simulink model "PD_Diagonal"  (R2015a)
settings: Solver=ode4  StartTime=0.0  StopTime=15  RelTol=1e-3
model workspace: external: MAT-File co-effs.mat (data not in the file)
undefined symbols (not defined in the file or in its folder): magnitude
libraries: aerolibutil x104, vrlib x5, dspmathops x4, simulink_extras x2, simulink x1, dspinverses x1
(part 2 of 3)

== system PD_Diagonal/M2/M2->B Transformation ==
  note: X->Y->Z Transformation Sequence M2->B
  X : Inport
  Y : Inport  Port=2
  "Z " : Inport  Port=3
  Quaternion Multiplication : aerolibutil/Quaternion Multiplication
  Quaternion Multiplication1 : aerolibutil/Quaternion Multiplication
  X Quaternion : Subsystem
  Y Quaternion : Subsystem
  Z Quaternion : Subsystem
  Q_m2 : Outport
  tag scope: M2x=global, M2y=global, M2z=global
  wires:
  X/1 -> X Quaternion/1(y(X Rad)), [M2x]
  "Z "/1 -> [M2z], Z Quaternion/1(Z Rad)
  Y/1 -> Y Quaternion/1(h(Y Rad)), [M2y]
  Y Quaternion/1(Q_y) -> Quaternion Multiplication/2  "Qy"
  X Quaternion/1(Q_x) -> Quaternion Multiplication/1  "Qx"
  Quaternion Multiplication/1 -> Quaternion Multiplication1/1  "Qx*Qy"
  Z Quaternion/1(Q_z) -> Quaternion Multiplication1/2  "Qz"
  Quaternion Multiplication1/1 -> Q_m2/1  "Qx*Qy*Qz"

== system PD_Diagonal/M3/M3 DC Motor ==
  note: M3 DC Motor response
  Set Speed(rpm) : Inport
  ->ms : Product  Inputs=*/
  10080 Max : Saturate  UpperLimit=10080  LowerLimit=-10080
  Add : Sum
  Dead Time (ms) : Constant
  Dead Time Block : VariableTransportDelay  MaximumDelay=10
  Miliseconds : Constant  Value=1000
  Starting Speed : Constant  Value=10080
  Subtract : Sum  Inputs=+-
  Transfer Fcn : TransferFcn  Numerator=1  Denominator=[0.6 1]
  Speed (rpm) : Outport
  wires:
  Dead Time Block/1 -> Transfer Fcn/1
  Miliseconds/1 -> ->ms/2
  Dead Time (ms)/1 -> ->ms/1
  ->ms/1 -> Dead Time Block/2
  Transfer Fcn/1 -> 10080 Max/1
  Set Speed(rpm)/1 -> Subtract/1
  10080 Max/1 -> Add/1
  Add/1 -> Speed (rpm)/1
  Starting Speed/1 -> Subtract/2, Add/2
  Subtract/1 -> Dead Time Block/1

== system PD_Diagonal/M3/M3 Speed to Thrust ==
  note: RPS to Thrust
  Speed(RPM) : Inport
  ->RPS : Product  Inputs=*/
  Force Coefficient CT : Constant  Value=0.000243
  M1 w^2 : Math  Operator=magnitude^2  SaturateOnIntegerOverflow=on
  Mins : Constant  Value=60
  Product : Product
  Thrust(N) : Outport
  wires:
  M1 w^2/1 -> Product/2
  ->RPS/1 -> M1 w^2/1
  Speed(RPM)/1 -> ->RPS/1
  Force Coefficient CT/1 -> Product/1
  Mins/1 -> ->RPS/2
  Product/1 -> Thrust(N)/1

== system PD_Diagonal/M3/M3 X Servo  ==
  note: 0V Servo = 0 degree / +90 offset
      | 2.5v Servo = 90 degree/ 0 offset
      | 5v Servo = 180 degree / -90 offset
  note: Servo zero position = 2.5v = 90 degree vertical
  note: 2.5v = 90 degree
  note: 2.5v = 0 offset
  note: M3X Servo Response v->rad
  Input(v) : Inport
  ->ms : Product  Inputs=*/
  ->rad : Constant  Value=pi/5
  Add : Sum  Inputs=+-
  Dead Time (ms) : Constant  Value=3
  Dead Time Block : VariableTransportDelay  MaximumDelay=10  MaximumPoints=2048
  Default Zero : Constant  Value=pi/2
  Divide : Product  Inputs=*/
  Miliseconds : Constant  Value=1000
  Multiply : Product  Inputs=**
  Saturation : Subsystem
  Scope : Scope
      settings: SaveName=ScopeData3
  Starting Position(v) : Constant  Value=2.5
  Subtract : Sum  Inputs=|-+
  Subtract1 : Sum  Inputs=+-|
  Supply (V) : Constant  Value=5
  Transfer Fcn : TransferFcn  Numerator=[pi]  Denominator=[0.11 1]
  Position (rad) : Outport
  wires:
  Miliseconds/1 -> ->ms/2
  Dead Time (ms)/1 -> ->ms/1
  Supply (V)/1 -> Divide/2
  Divide/1 -> Dead Time Block/1
  ->ms/1 -> Dead Time Block/2  "Deadtime 3ms (333hz digital)"
  Dead Time Block/1 -> Transfer Fcn/1
  ->rad/1 -> Multiply/2
  Transfer Fcn/1 -> Saturation/1(Rad)
  Saturation/1(Out1) -> Add/1
  [Lim] -> Saturation/2(1/0)
  Starting Position(v)/1 -> Multiply/1, Subtract/2
  Subtract/1 -> Divide/1
  Add/1 -> Scope/1, Position (rad)/1
  Multiply/1 -> Subtract1/2
  Input(v)/1 -> Subtract/1
  Subtract1/1 -> Add/2
  Default Zero/1 -> Subtract1/1

== system PD_Diagonal/M3/M3 Y Servo ==
  note: 0V Servo = 0 degree / +90 offset
      | 2.5v Servo = 90 degree/ 0 offset
      | 5v Servo = 180 degree / -90 offset
  note: Servo zero position = 2.5v = 90 degree vertical
  note: 2.5v = 90 degree
  note: 2.5v = 0 offset
  note: M3Y Servo Response v->rad
  Input(v) : Inport
  ->ms : Product  Inputs=*/
  ->rad : Constant  Value=pi/5
  Add : Sum  Inputs=+-
  Dead Time (ms) : Constant  Value=3
  Dead Time Block : VariableTransportDelay  MaximumDelay=10  MaximumPoints=2048
  Default Zero : Constant  Value=pi/2
  Divide : Product  Inputs=*/
  Miliseconds : Constant  Value=1000
  Multiply : Product  Inputs=**
  Saturation : Subsystem
  Scope : Scope
      settings: SaveName=ScopeData4
  Starting Position(v) : Constant  Value=2.5
  Subtract : Sum  Inputs=|-+
  Subtract1 : Sum  Inputs=+-|
  Supply (V) : Constant  Value=5
  Transfer Fcn : TransferFcn  Numerator=[pi]  Denominator=[0.11 1]
  Position (rad) : Outport
  wires:
  Miliseconds/1 -> ->ms/2
  Dead Time (ms)/1 -> ->ms/1
  Supply (V)/1 -> Divide/2
  Divide/1 -> Dead Time Block/1
  ->ms/1 -> Dead Time Block/2  "Deadtime 3ms (333hz digital)"
  Dead Time Block/1 -> Transfer Fcn/1
  ->rad/1 -> Multiply/2
  Transfer Fcn/1 -> Saturation/1(Rad)
  Saturation/1(Out1) -> Add/1
  [Lim] -> Saturation/2(1/0)
  Starting Position(v)/1 -> Multiply/1, Subtract/2
  Subtract/1 -> Divide/1
  Add/1 -> Scope/1, Position (rad)/1
  Multiply/1 -> Subtract1/2
  Input(v)/1 -> Subtract/1
  Subtract1/1 -> Add/2
  Default Zero/1 -> Subtract1/1

== system PD_Diagonal/M3/M3->B Transformation ==
  note: X->Y->Z Transformation Sequence M3->B
  X : Inport
  Y : Inport  Port=2
  "Z " : Inport  Port=3
  Quaternion Multiplication : aerolibutil/Quaternion Multiplication
  Quaternion Multiplication1 : aerolibutil/Quaternion Multiplication
  X Quaternion : Subsystem
  Y Quaternion : Subsystem
  Z Quaternion : Subsystem
  Q_m3 : Outport
  tag scope: M3x=global, M3y=global, M3z=global
  wires:
  X/1 -> X Quaternion/1(y(X Rad)), [M3x]
  "Z "/1 -> [M3z], Z Quaternion/1(Z Rad)
  Y/1 -> Y Quaternion/1(h(Y Rad)), [M3y]
  Y Quaternion/1(Q_y) -> Quaternion Multiplication/2  "Qy"
  X Quaternion/1(Q_x) -> Quaternion Multiplication/1  "Qx"
  Quaternion Multiplication/1 -> Quaternion Multiplication1/1  "Qx*Qy"
  Z Quaternion/1(Q_z) -> Quaternion Multiplication1/2  "Qz"
  Quaternion Multiplication1/1 -> Q_m3/1  "Qx*Qy*Qz"

== system PD_Diagonal/M4/M4 DC Motor ==
  note: M4 DC Motor response
  Set Speed(rpm) : Inport
  ->ms : Product  Inputs=*/
  10080 Max : Saturate  UpperLimit=10080  LowerLimit=-10080
  Add : Sum
  Dead Time (ms) : Constant
  Dead Time Block : VariableTransportDelay  MaximumDelay=10
  Miliseconds : Constant  Value=1000
  Starting Speed : Constant  Value=-10080
  Subtract : Sum  Inputs=+-
  Transfer Fcn : TransferFcn  Numerator=1  Denominator=[0.6 1]
  Speed (rpm) : Outport
  wires:
  Dead Time Block/1 -> Transfer Fcn/1
  Miliseconds/1 -> ->ms/2
  Dead Time (ms)/1 -> ->ms/1
  ->ms/1 -> Dead Time Block/2
  Transfer Fcn/1 -> 10080 Max/1
  Set Speed(rpm)/1 -> Subtract/1
  10080 Max/1 -> Add/1
  Add/1 -> Speed (rpm)/1
  Starting Speed/1 -> Subtract/2, Add/2
  Subtract/1 -> Dead Time Block/1

== system PD_Diagonal/M4/M4 Speed to Thrust ==
  note: RPS to Thrust
  Speed(RPM) : Inport
  ->RPS : Product  Inputs=*/
  Force Coefficient CT : Constant  Value=0.000243
  M1 w^2 : Math  Operator=magnitude^2  SaturateOnIntegerOverflow=on
  Mins : Constant  Value=60
  Product : Product
  Thrust(N) : Outport
  wires:
  M1 w^2/1 -> Product/2
  ->RPS/1 -> M1 w^2/1
  Speed(RPM)/1 -> ->RPS/1
  Force Coefficient CT/1 -> Product/1
  Mins/1 -> ->RPS/2
  Product/1 -> Thrust(N)/1

== system PD_Diagonal/M4/M4 X Servo  ==
  note: 0V Servo = 0 degree / +90 offset
      | 2.5v Servo = 90 degree/ 0 offset
      | 5v Servo = 180 degree / -90 offset
  note: Servo zero position = 2.5v = 90 degree vertical
  note: 2.5v = 90 degree
  note: 2.5v = 0 offset
  note: M4X Servo Response v->rad
  Input(v) : Inport
  ->ms : Product  Inputs=*/
  ->rad : Constant  Value=pi/5
  Add : Sum  Inputs=+-
  Dead Time (ms) : Constant  Value=3
  Dead Time Block : VariableTransportDelay  MaximumDelay=10  MaximumPoints=2048
  Default Zero : Constant  Value=pi/2
  Divide : Product  Inputs=*/
  Miliseconds : Constant  Value=1000
  Multiply : Product  Inputs=**
  Saturation : Subsystem
  Scope : Scope
      settings: SaveName=ScopeData3
  Starting Position(v) : Constant  Value=2.5
  Subtract : Sum  Inputs=|-+
  Subtract1 : Sum  Inputs=+-|
  Supply (V) : Constant  Value=5
  Transfer Fcn : TransferFcn  Numerator=[pi]  Denominator=[0.11 1]
  Position (rad) : Outport
  wires:
  Miliseconds/1 -> ->ms/2
  Dead Time (ms)/1 -> ->ms/1
  Supply (V)/1 -> Divide/2
  Divide/1 -> Dead Time Block/1
  ->ms/1 -> Dead Time Block/2  "Deadtime 3ms (333hz digital)"
  Dead Time Block/1 -> Transfer Fcn/1
  ->rad/1 -> Multiply/2
  Transfer Fcn/1 -> Saturation/1(Rad)
  Saturation/1(Out1) -> Add/1
  [Lim] -> Saturation/2(1/0)
  Starting Position(v)/1 -> Multiply/1, Subtract/2
  Subtract/1 -> Divide/1
  Add/1 -> Scope/1, Position (rad)/1
  Multiply/1 -> Subtract1/2
  Input(v)/1 -> Subtract/1
  Subtract1/1 -> Add/2
  Default Zero/1 -> Subtract1/1

== system PD_Diagonal/M4/M4 Y Servo ==
  note: 0V Servo = 0 degree / +90 offset
      | 2.5v Servo = 90 degree/ 0 offset
      | 5v Servo = 180 degree / -90 offset
  note: Servo zero position = 2.5v = 90 degree vertical
  note: 2.5v = 90 degree
  note: 2.5v = 0 offset
  note: M4Y Servo Response v->rad
  Input(v) : Inport
  ->ms : Product  Inputs=*/
  ->rad : Constant  Value=pi/5
  Add : Sum  Inputs=+-
  Dead Time (ms) : Constant  Value=3
  Dead Time Block : VariableTransportDelay  MaximumDelay=10  MaximumPoints=2048
  Default Zero : Constant  Value=pi/2
  Divide : Product  Inputs=*/
  Miliseconds : Constant  Value=1000
  Multiply : Product  Inputs=**
  Saturation : Subsystem
  Scope : Scope
      settings: SaveName=ScopeData4
  Starting Position(v) : Constant  Value=2.5
  Subtract : Sum  Inputs=|-+
  Subtract1 : Sum  Inputs=+-|
  Supply (V) : Constant  Value=5
  Transfer Fcn : TransferFcn  Numerator=[pi]  Denominator=[0.11 1]
  Position (rad) : Outport
  wires:
  Miliseconds/1 -> ->ms/2
  Dead Time (ms)/1 -> ->ms/1
  Supply (V)/1 -> Divide/2
  Divide/1 -> Dead Time Block/1
  ->ms/1 -> Dead Time Block/2  "Deadtime 3ms (333hz digital)"
  Dead Time Block/1 -> Transfer Fcn/1
  ->rad/1 -> Multiply/2
  Transfer Fcn/1 -> Saturation/1(Rad)
  Saturation/1(Out1) -> Add/1
  [Lim] -> Saturation/2(1/0)
  Starting Position(v)/1 -> Multiply/1, Subtract/2
  Subtract/1 -> Divide/1
  Add/1 -> Scope/1, Position (rad)/1
  Multiply/1 -> Subtract1/2
  Input(v)/1 -> Subtract/1
  Subtract1/1 -> Add/2
  Default Zero/1 -> Subtract1/1

== system PD_Diagonal/M4/M4->B Transformation ==
  note: X->Y->Z Transformation Sequence M4->B
  X : Inport
  Y : Inport  Port=2
  "Z " : Inport  Port=3
  Quaternion Multiplication : aerolibutil/Quaternion Multiplication
  Quaternion Multiplication1 : aerolibutil/Quaternion Multiplication
  X Quaternion : Subsystem
  Y Quaternion : Subsystem
  Z Quaternion : Subsystem
  Q_m4 : Outport
  tag scope: M4x=global, M4y=global, M4z=global
  wires:
  X/1 -> X Quaternion/1(y(X Rad)), [M4x]
  Y/1 -> Y Quaternion/1(h(Y Rad)), [M4y]
  Y Quaternion/1(Q_y) -> Quaternion Multiplication/2  "Qy"
  X Quaternion/1(Q_x) -> Quaternion Multiplication/1  "Qx"
  Quaternion Multiplication/1 -> Quaternion Multiplication1/1  "Qx*Qy"
  Z Quaternion/1(Q_z) -> Quaternion Multiplication1/2  "Qz"
  Quaternion Multiplication1/1 -> Q_m4/1  "Qx*Qy*Qz"
  "Z "/1 -> [M4z], Z Quaternion/1(Z Rad)

== system PD_Diagonal/Quat Error/QuatMultiply1 ==
  Q1 in : Inport  PortDimensions=[4]
  Q2 in : Inport  Port=2  PortDimensions=[4]
  Q1 scalar : Selector  InputPortWidth=4  Indices=[1]
  Q1 vector : Selector  InputPortWidth=4  Indices=[2 3 4]
  Q1.Q2 : DotProduct  InputSameDT=on  OutDataTypeStr=Inherit: Inherit via internal rule
  Q1XQ2 : vrlib/Utilities/Cross Product
  Q2 scalar : Selector  InputPortWidth=4  Indices=[1]
  Q2 vector : Selector  InputPortWidth=4  Indices=[2 3 4]
  Qout scalar : Sum  Inputs=+-
  Qout vector : Sum  Inputs=+++
  Vector Concatenate : Concatenate
  q1.Q2 : Product
  q1.q2 : Product
  q2.Q1 : Product
  Qout : Outport  PortDimensions=[4]
  wires:
  Q1 in/1 -> Q1 vector/1, Q1 scalar/1
  Q2 in/1 -> Q2 vector/1, Q2 scalar/1
  Q1 scalar/1 -> q1.q2/1, q1.Q2/1
  Q2 scalar/1 -> q1.q2/2, q2.Q1/2
  Q1 vector/1 -> Q1.Q2/1, Q1XQ2/1, q2.Q1/1
  Q2 vector/1 -> Q1.Q2/2, Q1XQ2/2, q1.Q2/2
  q1.q2/1 -> Qout scalar/1
  Q1.Q2/1 -> Qout scalar/2
  q2.Q1/1 -> Qout vector/1
  q1.Q2/1 -> Qout vector/2
  Qout scalar/1 -> Vector Concatenate/1
  Qout vector/1 -> Vector Concatenate/2
  Vector Concatenate/1 -> Qout/1
  Q1XQ2/1 -> Qout vector/3  "Q1XQ2"

== system PD_Diagonal/R->Q/QuatMultiply ==
  Q1 in : Inport  PortDimensions=[4]
  Q2 in : Inport  Port=2  PortDimensions=[4]
  Q1 scalar : Selector  InputPortWidth=4  Indices=[1]
  Q1 vector : Selector  InputPortWidth=4  Indices=[2 3 4]
  Q1.Q2 : DotProduct  InputSameDT=on  OutDataTypeStr=Inherit: Inherit via internal rule
  Q1XQ2 : vrlib/Utilities/Cross Product
  Q2 scalar : Selector  InputPortWidth=4  Indices=[1]
  Q2 vector : Selector  InputPortWidth=4  Indices=[2 3 4]
  Qout scalar : Sum  Inputs=+-
  Qout vector : Sum  Inputs=+++
  Vector Concatenate : Concatenate
  q1.Q2 : Product
  q1.q2 : Product
  q2.Q1 : Product
  Qout : Outport  PortDimensions=[4]
  wires:
  Q1 in/1 -> Q1 vector/1, Q1 scalar/1
  Q2 in/1 -> Q2 vector/1, Q2 scalar/1
  Q1 scalar/1 -> q1.q2/1, q1.Q2/1
  Q2 scalar/1 -> q1.q2/2, q2.Q1/2
  Q1 vector/1 -> Q1.Q2/1, q2.Q1/1, Q1XQ2/1
  Q2 vector/1 -> Q1.Q2/2, q1.Q2/2, Q1XQ2/2
  q1.q2/1 -> Qout scalar/1
  Q1.Q2/1 -> Qout scalar/2
  q2.Q1/1 -> Qout vector/1
  q1.Q2/1 -> Qout vector/2
  Q1XQ2/1 -> Qout vector/3
  Qout scalar/1 -> Vector Concatenate/1
  Qout vector/1 -> Vector Concatenate/2
  Vector Concatenate/1 -> Qout/1

== system PD_Diagonal/R->Q/QuatMultiply1 ==
  Q1 in : Inport  PortDimensions=[4]
  Q2 in : Inport  Port=2  PortDimensions=[4]
  Q1 scalar : Selector  InputPortWidth=4  Indices=[1]
  Q1 vector : Selector  InputPortWidth=4  Indices=[2 3 4]
  Q1.Q2 : DotProduct  InputSameDT=on  OutDataTypeStr=Inherit: Inherit via internal rule
  Q1XQ2 : vrlib/Utilities/Cross Product
  Q2 scalar : Selector  InputPortWidth=4  Indices=[1]
  Q2 vector : Selector  InputPortWidth=4  Indices=[2 3 4]
  Qout scalar : Sum  Inputs=+-
  Qout vector : Sum  Inputs=+++
  Vector Concatenate : Concatenate
  q1.Q2 : Product
  q1.q2 : Product
  q2.Q1 : Product
  Qout : Outport  PortDimensions=[4]
  wires:
  Q1 in/1 -> Q1 vector/1, Q1 scalar/1
  Q2 in/1 -> Q2 vector/1, Q2 scalar/1
  Q1 scalar/1 -> q1.q2/1, q1.Q2/1
  Q2 scalar/1 -> q1.q2/2, q2.Q1/2
  Q1 vector/1 -> Q1.Q2/1, Q1XQ2/1, q2.Q1/1
  Q2 vector/1 -> Q1.Q2/2, Q1XQ2/2, q1.Q2/2
  q1.q2/1 -> Qout scalar/1
  Q1.Q2/1 -> Qout scalar/2
  q2.Q1/1 -> Qout vector/1
  q1.Q2/1 -> Qout vector/2
  Qout scalar/1 -> Vector Concatenate/1
  Qout vector/1 -> Vector Concatenate/2
  Vector Concatenate/1 -> Qout/1
  Q1XQ2/1 -> Qout vector/3  "Q1XQ2"

== system PD_Diagonal/Rb0->Q0/QuatMultiply ==
  Q1 in : Inport  PortDimensions=[4]
  Q2 in : Inport  Port=2  PortDimensions=[4]
  Q1 scalar : Selector  InputPortWidth=4  Indices=[1]
  Q1 vector : Selector  InputPortWidth=4  Indices=[2 3 4]
  Q1.Q2 : DotProduct  InputSameDT=on  OutDataTypeStr=Inherit: Inherit via internal rule
  Q1XQ2 : vrlib/Utilities/Cross Product
  Q2 scalar : Selector  InputPortWidth=4  Indices=[1]
  Q2 vector : Selector  InputPortWidth=4  Indices=[2 3 4]
  Qout scalar : Sum  Inputs=+-
  Qout vector : Sum  Inputs=+++
  Vector Concatenate : Concatenate
  q1.Q2 : Product
  q1.q2 : Product
  q2.Q1 : Product
  Qout : Outport  PortDimensions=[4]
  wires:
  Q1 in/1 -> Q1 vector/1, Q1 scalar/1
  Q2 in/1 -> Q2 vector/1, Q2 scalar/1
  Q1 scalar/1 -> q1.q2/1, q1.Q2/1
  Q2 scalar/1 -> q1.q2/2, q2.Q1/2
  Q1 vector/1 -> Q1.Q2/1, q2.Q1/1, Q1XQ2/1
  Q2 vector/1 -> Q1.Q2/2, q1.Q2/2, Q1XQ2/2
  q1.q2/1 -> Qout scalar/1
  Q1.Q2/1 -> Qout scalar/2
  q2.Q1/1 -> Qout vector/1
  q1.Q2/1 -> Qout vector/2
  Q1XQ2/1 -> Qout vector/3
  Qout scalar/1 -> Vector Concatenate/1
  Qout vector/1 -> Vector Concatenate/2
  Vector Concatenate/1 -> Qout/1

== system PD_Diagonal/Rb0->Q0/QuatMultiply1 ==
  Q1 in : Inport  PortDimensions=[4]
  Q2 in : Inport  Port=2  PortDimensions=[4]
  Q1 scalar : Selector  InputPortWidth=4  Indices=[1]
  Q1 vector : Selector  InputPortWidth=4  Indices=[2 3 4]
  Q1.Q2 : DotProduct  InputSameDT=on  OutDataTypeStr=Inherit: Inherit via internal rule
  Q1XQ2 : vrlib/Utilities/Cross Product
  Q2 scalar : Selector  InputPortWidth=4  Indices=[1]
  Q2 vector : Selector  InputPortWidth=4  Indices=[2 3 4]
  Qout scalar : Sum  Inputs=+-
  Qout vector : Sum  Inputs=+++
  Vector Concatenate : Concatenate
  q1.Q2 : Product
  q1.q2 : Product
  q2.Q1 : Product
  Qout : Outport  PortDimensions=[4]
  wires:
  Q1 in/1 -> Q1 vector/1, Q1 scalar/1
  Q2 in/1 -> Q2 vector/1, Q2 scalar/1
  Q1 scalar/1 -> q1.q2/1, q1.Q2/1
  Q2 scalar/1 -> q1.q2/2, q2.Q1/2
  Q1 vector/1 -> Q1.Q2/1, Q1XQ2/1, q2.Q1/1
  Q2 vector/1 -> Q1.Q2/2, Q1XQ2/2, q1.Q2/2
  q1.q2/1 -> Qout scalar/1
  Q1.Q2/1 -> Qout scalar/2
  q2.Q1/1 -> Qout vector/1
  q1.Q2/1 -> Qout vector/2
  Qout scalar/1 -> Vector Concatenate/1
  Qout vector/1 -> Vector Concatenate/2
  Vector Concatenate/1 -> Qout/1
  Q1XQ2/1 -> Qout vector/3  "Q1XQ2"

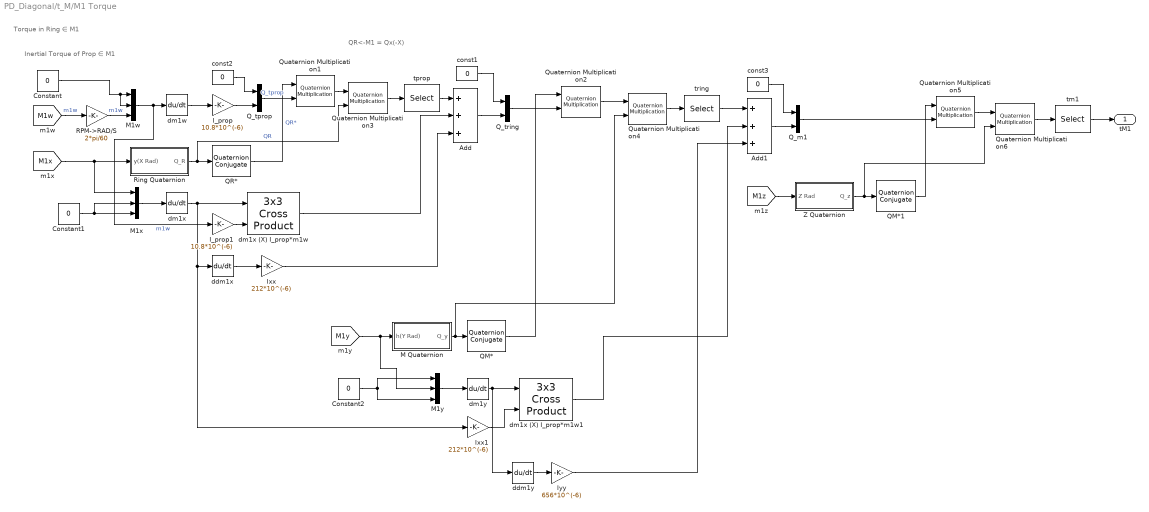
== system PD_Diagonal/t_M/M1 Torque ==
  note: QR<-M1 = Qx(-X)
  note: Torque in Ring ∈ M1
  note: Inertial Torque of Prop ∈ M1
  Add : Sum  Inputs=+++
  Add1 : Sum  Inputs=+++
  Constant : Constant  Value=0
  Constant1 : Constant  Value=0
  Constant2 : Constant  Value=0
  I_prop : Gain  Gain=10.8*10^(-6)
  I_prop1 : Gain  Gain=10.8*10^(-6)
  Ixx : Gain  Gain=212*10^(-6)
  Ixx1 : Gain  Gain=212*10^(-6)
  Iyy : Gain  Gain=656*10^(-6)
  M Quaternion : Subsystem
  M1w : Concatenate  NumInputs=3
  M1x : Concatenate  NumInputs=3
  M1y : Concatenate  NumInputs=3
  QM* : aerolibutil/Quaternion Conjugate
  QM*1 : aerolibutil/Quaternion Conjugate
  QR* : aerolibutil/Quaternion Conjugate
  Q_m1 : Concatenate
  Q_tprop : Concatenate
  Q_tring : Concatenate
  Quaternion Multiplication{1..6} (6 alike) : aerolibutil/Quaternion Multiplication
  RPM->RAD/S : Gain  Gain=2*pi/60
  Ring Quaternion : Subsystem
  Z Quaternion : Subsystem
  const1 : Constant  Value=0
  const2 : Constant  Value=0
  const3 : Constant  Value=0
  ddm1x : Derivative
  ddm1y : Derivative
  dm1w : Derivative
  dm1x : Derivative
  dm1x (X) I_prop*m1w : aerolibutil/3x3 Cross Product
  dm1x (X) I_prop*m1w1 : aerolibutil/3x3 Cross Product
  dm1y : Derivative
  tm1 : Selector  InputPortWidth=4  Indices=[2 3 4]
  tprop : Selector  InputPortWidth=4  Indices=[2 3 4]
  tring : Selector  InputPortWidth=4  Indices=[2 3 4]
  tM1 : Outport
  wires:
  [M1w] -> RPM->RAD/S/1  "m1w"
  RPM->RAD/S/1 -> M1w/3  "m1w"
  Constant/1 -> M1w/2, M1w/1
  dm1w/1 -> I_prop/1
  [M1x] -> M1x/1, Ring Quaternion/1(y(X Rad))
  Ring Quaternion/1(Q_R) -> Quaternion Multiplication3/2, QR*/1  "QR"
  const2/1 -> Q_tprop/1
  Quaternion Multiplication1/1 -> Quaternion Multiplication3/1
  Q_tprop/1 -> Quaternion Multiplication1/2  "Q_tprop"
  QR*/1 -> Quaternion Multiplication1/1  "QR*"
  I_prop/1 -> Q_tprop/2
  dm1x/1 -> Ixx1/1, ddm1x/1, dm1x (X) I_prop*m1w/1
  I_prop1/1 -> dm1x (X) I_prop*m1w/2
  dm1x (X) I_prop*m1w/1 -> Add/2
  M1w/1 -> I_prop1/1, dm1w/1  "m1w"
  M1x/1 -> dm1x/1
  ddm1x/1 -> Ixx/1
  Ixx/1 -> Add/3
  Quaternion Multiplication3/1 -> tprop/1
  tprop/1 -> Add/1
  [M1y] -> M1y/2, M Quaternion/1(h(Y Rad))
  const1/1 -> Q_tring/1
  Add/1 -> Q_tring/2
  Q_tring/1 -> Quaternion Multiplication2/2
  M Quaternion/1(Q_y) -> Quaternion Multiplication4/2, QM*/1
  QM*/1 -> Quaternion Multiplication2/1
  Quaternion Multiplication2/1 -> Quaternion Multiplication4/1
  Quaternion Multiplication4/1 -> tring/1
  tring/1 -> Add1/1
  Constant1/1 -> M1x/2, M1x/3
  Constant2/1 -> M1y/1, M1y/3
  M1y/1 -> dm1y/1
  Ixx1/1 -> dm1x (X) I_prop*m1w1/2
  dm1x (X) I_prop*m1w1/1 -> Add1/2
  dm1y/1 -> ddm1y/1, dm1x (X) I_prop*m1w1/1
  ddm1y/1 -> Iyy/1
  Iyy/1 -> Add1/3
  [M1z] -> Z Quaternion/1(Z Rad)
  const3/1 -> Q_m1/1
  Add1/1 -> Q_m1/2
  Q_m1/1 -> Quaternion Multiplication5/2
  Z Quaternion/1(Q_z) -> Quaternion Multiplication6/2, QM*1/1
  QM*1/1 -> Quaternion Multiplication5/1
  Quaternion Multiplication5/1 -> Quaternion Multiplication6/1
  Quaternion Multiplication6/1 -> tm1/1
  tm1/1 -> tM1/1

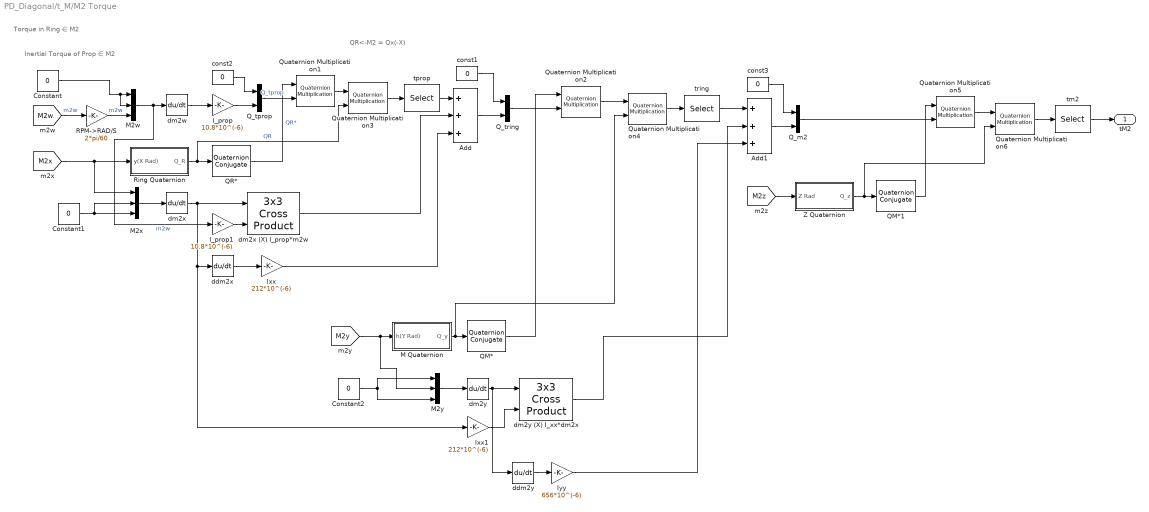
== system PD_Diagonal/t_M/M2 Torque ==
  note: QR<-M2 = Qx(-X)
  note: Torque in Ring ∈ M2
  note: Inertial Torque of Prop ∈ M2
  Add : Sum  Inputs=+++
  Add1 : Sum  Inputs=+++
  Constant : Constant  Value=0
  Constant1 : Constant  Value=0
  Constant2 : Constant  Value=0
  I_prop : Gain  Gain=10.8*10^(-6)
  I_prop1 : Gain  Gain=10.8*10^(-6)
  Ixx : Gain  Gain=212*10^(-6)
  Ixx1 : Gain  Gain=212*10^(-6)
  Iyy : Gain  Gain=656*10^(-6)
  M Quaternion : Subsystem
  M2w : Concatenate  NumInputs=3
  M2x : Concatenate  NumInputs=3
  M2y : Concatenate  NumInputs=3
  QM* : aerolibutil/Quaternion Conjugate
  QM*1 : aerolibutil/Quaternion Conjugate
  QR* : aerolibutil/Quaternion Conjugate
  Q_m2 : Concatenate
  Q_tprop : Concatenate
  Q_tring : Concatenate
  Quaternion Multiplication{1..6} (6 alike) : aerolibutil/Quaternion Multiplication
  RPM->RAD/S : Gain  Gain=2*pi/60
  Ring Quaternion : Subsystem
  Z Quaternion : Subsystem
  const1 : Constant  Value=0
  const2 : Constant  Value=0
  const3 : Constant  Value=0
  ddm2x : Derivative
  ddm2y : Derivative
  dm2w : Derivative
  dm2x : Derivative
  dm2x (X) I_prop*m2w : aerolibutil/3x3 Cross Product
  dm2y : Derivative
  dm2y (X) I_xx*dm2x : aerolibutil/3x3 Cross Product
  tm2 : Selector  InputPortWidth=4  Indices=[2 3 4]
  tprop : Selector  InputPortWidth=4  Indices=[2 3 4]
  tring : Selector  InputPortWidth=4  Indices=[2 3 4]
  tM2 : Outport
  wires:
  [M2w] -> RPM->RAD/S/1  "m2w"
  RPM->RAD/S/1 -> M2w/3  "m2w"
  Constant/1 -> M2w/2, M2w/1
  dm2w/1 -> I_prop/1
  [M2x] -> M2x/1, Ring Quaternion/1(y(X Rad))
  Ring Quaternion/1(Q_R) -> Quaternion Multiplication3/2, QR*/1  "QR"
  const2/1 -> Q_tprop/1
  Quaternion Multiplication1/1 -> Quaternion Multiplication3/1
  Q_tprop/1 -> Quaternion Multiplication1/2  "Q_tprop"
  QR*/1 -> Quaternion Multiplication1/1  "QR*"
  I_prop/1 -> Q_tprop/2
  dm2x/1 -> Ixx1/1, ddm2x/1, dm2x (X) I_prop*m2w/1
  I_prop1/1 -> dm2x (X) I_prop*m2w/2
  dm2x (X) I_prop*m2w/1 -> Add/2
  M2w/1 -> I_prop1/1, dm2w/1  "m2w"
  M2x/1 -> dm2x/1
  ddm2x/1 -> Ixx/1
  Ixx/1 -> Add/3
  Quaternion Multiplication3/1 -> tprop/1
  tprop/1 -> Add/1
  [M2y] -> M2y/2, M Quaternion/1(h(Y Rad))
  const1/1 -> Q_tring/1
  Add/1 -> Q_tring/2
  Q_tring/1 -> Quaternion Multiplication2/2
  M Quaternion/1(Q_y) -> Quaternion Multiplication4/2, QM*/1
  QM*/1 -> Quaternion Multiplication2/1
  Quaternion Multiplication2/1 -> Quaternion Multiplication4/1
  Quaternion Multiplication4/1 -> tring/1
  tring/1 -> Add1/1
  Constant1/1 -> M2x/2, M2x/3
  Constant2/1 -> M2y/1, M2y/3
  M2y/1 -> dm2y/1
  Ixx1/1 -> dm2y (X) I_xx*dm2x/2
  dm2y (X) I_xx*dm2x/1 -> Add1/2
  dm2y/1 -> ddm2y/1, dm2y (X) I_xx*dm2x/1
  ddm2y/1 -> Iyy/1
  Iyy/1 -> Add1/3
  [M2z] -> Z Quaternion/1(Z Rad)
  const3/1 -> Q_m2/1
  Add1/1 -> Q_m2/2
  Q_m2/1 -> Quaternion Multiplication5/2
  Z Quaternion/1(Q_z) -> Quaternion Multiplication6/2, QM*1/1
  QM*1/1 -> Quaternion Multiplication5/1
  Quaternion Multiplication5/1 -> Quaternion Multiplication6/1
  Quaternion Multiplication6/1 -> tm2/1
  tm2/1 -> tM2/1

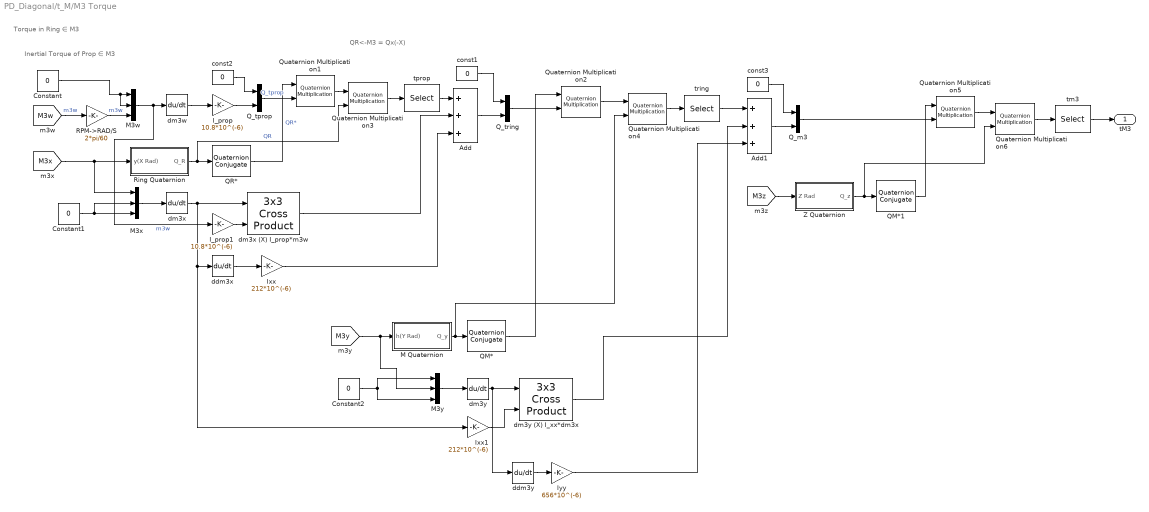
== system PD_Diagonal/t_M/M3 Torque ==
  note: QR<-M3 = Qx(-X)
  note: Torque in Ring ∈ M3
  note: Inertial Torque of Prop ∈ M3
  Add : Sum  Inputs=+++
  Add1 : Sum  Inputs=+++
  Constant : Constant  Value=0
  Constant1 : Constant  Value=0
  Constant2 : Constant  Value=0
  I_prop : Gain  Gain=10.8*10^(-6)
  I_prop1 : Gain  Gain=10.8*10^(-6)
  Ixx : Gain  Gain=212*10^(-6)
  Ixx1 : Gain  Gain=212*10^(-6)
  Iyy : Gain  Gain=656*10^(-6)
  M Quaternion : Subsystem
  M3w : Concatenate  NumInputs=3
  M3x : Concatenate  NumInputs=3
  M3y : Concatenate  NumInputs=3
  QM* : aerolibutil/Quaternion Conjugate
  QM*1 : aerolibutil/Quaternion Conjugate
  QR* : aerolibutil/Quaternion Conjugate
  Q_m3 : Concatenate
  Q_tprop : Concatenate
  Q_tring : Concatenate
  Quaternion Multiplication{1..6} (6 alike) : aerolibutil/Quaternion Multiplication
  RPM->RAD/S : Gain  Gain=2*pi/60
  Ring Quaternion : Subsystem
  Z Quaternion : Subsystem
  const1 : Constant  Value=0
  const2 : Constant  Value=0
  const3 : Constant  Value=0
  ddm3x : Derivative
  ddm3y : Derivative
  dm3w : Derivative
  dm3x : Derivative
  dm3x (X) I_prop*m3w : aerolibutil/3x3 Cross Product
  dm3y : Derivative
  dm3y (X) I_xx*dm3x : aerolibutil/3x3 Cross Product
  tm3 : Selector  InputPortWidth=4  Indices=[2 3 4]
  tprop : Selector  InputPortWidth=4  Indices=[2 3 4]
  tring : Selector  InputPortWidth=4  Indices=[2 3 4]
  tM3 : Outport
  wires:
  [M3w] -> RPM->RAD/S/1  "m3w"
  RPM->RAD/S/1 -> M3w/3  "m3w"
  Constant/1 -> M3w/2, M3w/1
  dm3w/1 -> I_prop/1
  [M3x] -> M3x/1, Ring Quaternion/1(y(X Rad))
  Ring Quaternion/1(Q_R) -> Quaternion Multiplication3/2, QR*/1  "QR"
  const2/1 -> Q_tprop/1
  Quaternion Multiplication1/1 -> Quaternion Multiplication3/1
  Q_tprop/1 -> Quaternion Multiplication1/2  "Q_tprop"
  QR*/1 -> Quaternion Multiplication1/1  "QR*"
  I_prop/1 -> Q_tprop/2
  dm3x/1 -> Ixx1/1, ddm3x/1, dm3x (X) I_prop*m3w/1
  I_prop1/1 -> dm3x (X) I_prop*m3w/2
  dm3x (X) I_prop*m3w/1 -> Add/2
  M3w/1 -> I_prop1/1, dm3w/1  "m3w"
  M3x/1 -> dm3x/1
  ddm3x/1 -> Ixx/1
  Ixx/1 -> Add/3
  Quaternion Multiplication3/1 -> tprop/1
  tprop/1 -> Add/1
  [M3y] -> M3y/2, M Quaternion/1(h(Y Rad))
  const1/1 -> Q_tring/1
  Add/1 -> Q_tring/2
  Q_tring/1 -> Quaternion Multiplication2/2
  M Quaternion/1(Q_y) -> Quaternion Multiplication4/2, QM*/1
  QM*/1 -> Quaternion Multiplication2/1
  Quaternion Multiplication2/1 -> Quaternion Multiplication4/1
  Quaternion Multiplication4/1 -> tring/1
  tring/1 -> Add1/1
  Constant1/1 -> M3x/2, M3x/3
  Constant2/1 -> M3y/1, M3y/3
  M3y/1 -> dm3y/1
  Ixx1/1 -> dm3y (X) I_xx*dm3x/2
  dm3y (X) I_xx*dm3x/1 -> Add1/2
  dm3y/1 -> ddm3y/1, dm3y (X) I_xx*dm3x/1
  ddm3y/1 -> Iyy/1
  Iyy/1 -> Add1/3
  [M3z] -> Z Quaternion/1(Z Rad)
  const3/1 -> Q_m3/1
  Add1/1 -> Q_m3/2
  Q_m3/1 -> Quaternion Multiplication5/2
  Z Quaternion/1(Q_z) -> Quaternion Multiplication6/2, QM*1/1
  QM*1/1 -> Quaternion Multiplication5/1
  Quaternion Multiplication5/1 -> Quaternion Multiplication6/1
  Quaternion Multiplication6/1 -> tm3/1
  tm3/1 -> tM3/1

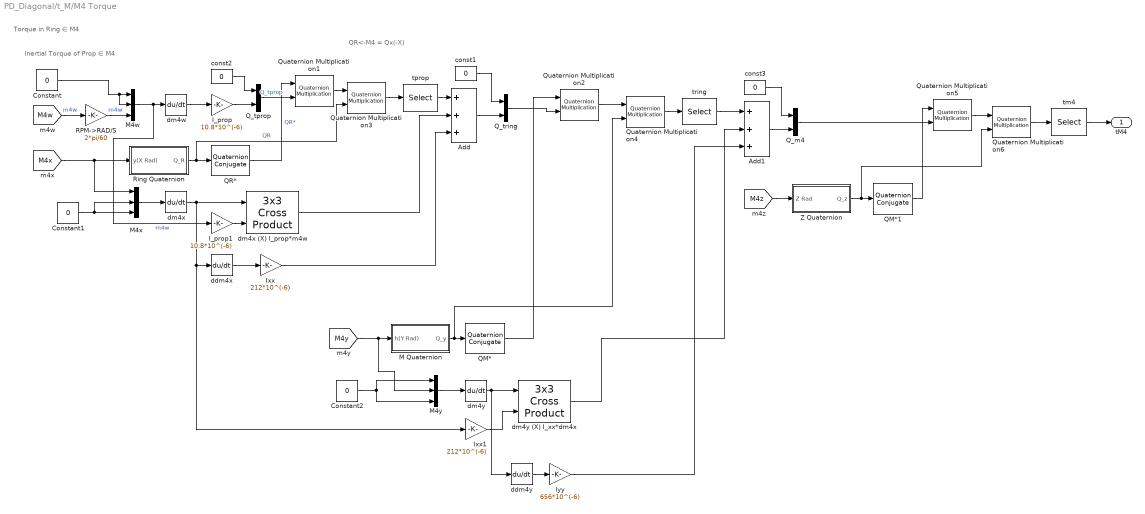
== system PD_Diagonal/t_M/M4 Torque ==
  note: QR<-M4 = Qx(-X)
  note: Torque in Ring ∈ M4
  note: Inertial Torque of Prop ∈ M4
  Add : Sum  Inputs=+++
  Add1 : Sum  Inputs=+++
  Constant : Constant  Value=0
  Constant1 : Constant  Value=0
  Constant2 : Constant  Value=0
  I_prop : Gain  Gain=10.8*10^(-6)
  I_prop1 : Gain  Gain=10.8*10^(-6)
  Ixx : Gain  Gain=212*10^(-6)
  Ixx1 : Gain  Gain=212*10^(-6)
  Iyy : Gain  Gain=656*10^(-6)
  M Quaternion : Subsystem
  M4w : Concatenate  NumInputs=3
  M4x : Concatenate  NumInputs=3
  M4y : Concatenate  NumInputs=3
  QM* : aerolibutil/Quaternion Conjugate
  QM*1 : aerolibutil/Quaternion Conjugate
  QR* : aerolibutil/Quaternion Conjugate
  Q_m4 : Concatenate
  Q_tprop : Concatenate
  Q_tring : Concatenate
  Quaternion Multiplication{1..6} (6 alike) : aerolibutil/Quaternion Multiplication
  RPM->RAD/S : Gain  Gain=2*pi/60
  Ring Quaternion : Subsystem
  Z Quaternion : Subsystem
  const1 : Constant  Value=0
  const2 : Constant  Value=0
  const3 : Constant  Value=0
  ddm4x : Derivative
  ddm4y : Derivative
  dm4w : Derivative
  dm4x : Derivative
  dm4x (X) I_prop*m4w : aerolibutil/3x3 Cross Product
  dm4y : Derivative
  dm4y (X) I_xx*dm4x : aerolibutil/3x3 Cross Product
  tm4 : Selector  InputPortWidth=4  Indices=[2 3 4]
  tprop : Selector  InputPortWidth=4  Indices=[2 3 4]
  tring : Selector  InputPortWidth=4  Indices=[2 3 4]
  tM4 : Outport
  wires:
  [M4w] -> RPM->RAD/S/1  "m4w"
  RPM->RAD/S/1 -> M4w/3  "m4w"
  Constant/1 -> M4w/2, M4w/1
  dm4w/1 -> I_prop/1
  [M4x] -> M4x/1, Ring Quaternion/1(y(X Rad))
  Ring Quaternion/1(Q_R) -> Quaternion Multiplication3/2, QR*/1  "QR"
  const2/1 -> Q_tprop/1
  Quaternion Multiplication1/1 -> Quaternion Multiplication3/1
  Q_tprop/1 -> Quaternion Multiplication1/2  "Q_tprop"
  QR*/1 -> Quaternion Multiplication1/1  "QR*"
  I_prop/1 -> Q_tprop/2
  dm4x/1 -> Ixx1/1, ddm4x/1, dm4x (X) I_prop*m4w/1
  I_prop1/1 -> dm4x (X) I_prop*m4w/2
  dm4x (X) I_prop*m4w/1 -> Add/2
  M4w/1 -> I_prop1/1, dm4w/1  "m4w"
  M4x/1 -> dm4x/1
  ddm4x/1 -> Ixx/1
  Ixx/1 -> Add/3
  Quaternion Multiplication3/1 -> tprop/1
  tprop/1 -> Add/1
  [M4y] -> M4y/2, M Quaternion/1(h(Y Rad))
  const1/1 -> Q_tring/1
  Add/1 -> Q_tring/2
  Q_tring/1 -> Quaternion Multiplication2/2
  M Quaternion/1(Q_y) -> Quaternion Multiplication4/2, QM*/1
  QM*/1 -> Quaternion Multiplication2/1
  Quaternion Multiplication2/1 -> Quaternion Multiplication4/1
  Quaternion Multiplication4/1 -> tring/1
  tring/1 -> Add1/1
  Constant1/1 -> M4x/2, M4x/3
  Constant2/1 -> M4y/1, M4y/3
  M4y/1 -> dm4y/1
  Ixx1/1 -> dm4y (X) I_xx*dm4x/2
  dm4y (X) I_xx*dm4x/1 -> Add1/2
  dm4y/1 -> ddm4y/1, dm4y (X) I_xx*dm4x/1
  ddm4y/1 -> Iyy/1
  Iyy/1 -> Add1/3
  [M4z] -> Z Quaternion/1(Z Rad)
  const3/1 -> Q_m4/1
  Add1/1 -> Q_m4/2
  Q_m4/1 -> Quaternion Multiplication5/2
  Z Quaternion/1(Q_z) -> Quaternion Multiplication6/2, QM*1/1
  QM*1/1 -> Quaternion Multiplication5/1
  Quaternion Multiplication5/1 -> Quaternion Multiplication6/1
  Quaternion Multiplication6/1 -> tm4/1
  tm4/1 -> tM4/1

== system PD_Diagonal/Control Allocation/M1/M1 DC Motor ==
  note: M1 DC Motor response
  Set Speed(rpm) : Inport
  ->ms : Product  Inputs=*/
  10080 Max : Saturate  UpperLimit=10080  LowerLimit=-10080
  Add : Sum
  Dead Time (ms) : Constant
  Dead Time Block : VariableTransportDelay  MaximumDelay=10
  Miliseconds : Constant  Value=1000
  Starting Speed : Constant  Value=10080
  Subtract : Sum  Inputs=+-
  Transfer Fcn : TransferFcn  Numerator=1  Denominator=[0.6 1]
  Speed (rpm) : Outport
  wires:
  Dead Time Block/1 -> Transfer Fcn/1
  Miliseconds/1 -> ->ms/2
  Dead Time (ms)/1 -> ->ms/1
  ->ms/1 -> Dead Time Block/2
  Transfer Fcn/1 -> 10080 Max/1
  Set Speed(rpm)/1 -> Subtract/1
  10080 Max/1 -> Add/1
  Add/1 -> Speed (rpm)/1
  Starting Speed/1 -> Subtract/2, Add/2
  Subtract/1 -> Dead Time Block/1

== system PD_Diagonal/Control Allocation/M1/M1 Speed to Thrust ==
  note: RPS to Thrust
  Speed(RPM) : Inport
  ->RPS : Product  Inputs=*/
  Force Coefficient CT : Constant  Value=0.000243
  M1 w^2 : Math  Operator=magnitude^2  SaturateOnIntegerOverflow=on
  Mins : Constant  Value=60
  Product : Product
  Thrust(N) : Outport
  wires:
  M1 w^2/1 -> Product/2
  ->RPS/1 -> M1 w^2/1
  Speed(RPM)/1 -> ->RPS/1
  Force Coefficient CT/1 -> Product/1
  Mins/1 -> ->RPS/2
  Product/1 -> Thrust(N)/1

== system PD_Diagonal/Control Allocation/M1/M1 X Servo  ==
  note: 0V Servo = 0 degree / +90 offset
      | 2.5v Servo = 90 degree/ 0 offset
      | 5v Servo = 180 degree / -90 offset
  note: Servo zero position = 2.5v = 90 degree vertical
  note: 2.5v = 90 degree
  note: 2.5v = 0 offset
  note: M1X Servo Response v->rad
  Input(v) : Inport
  ->ms : Product  Inputs=*/
  ->rad : Constant  Value=pi/5
  Add : Sum  Inputs=+-
  Dead Time (ms) : Constant  Value=3
  Dead Time Block : VariableTransportDelay  MaximumDelay=10
  Default Zero : Constant  Value=pi/2
  Divide : Product  Inputs=*/
  Limits : Constant  OutDataTypeStr=boolean
  Miliseconds : Constant  Value=1000
  Multiply : Product  Inputs=**
  Saturation : Subsystem
  Scope : Scope
      settings: SaveName=ScopeData3
  Starting Position(v) : Constant  Value=2.5
  Subtract : Sum  Inputs=|-+
  Subtract1 : Sum  Inputs=+-|
  Supply (V) : Constant  Value=5
  Transfer Fcn : TransferFcn  Numerator=[pi]  Denominator=[0.11 1]
  Position (rad) : Outport
  wires:
  Miliseconds/1 -> ->ms/2
  Dead Time (ms)/1 -> ->ms/1
  Supply (V)/1 -> Divide/2
  Divide/1 -> Dead Time Block/1
  ->ms/1 -> Dead Time Block/2  "Deadtime 3ms (333hz digital)"
  Dead Time Block/1 -> Transfer Fcn/1
  ->rad/1 -> Multiply/2
  Transfer Fcn/1 -> Saturation/1(Rad)
  Saturation/1(Out1) -> Add/1
  Limits/1 -> Saturation/2(1/0)
  Starting Position(v)/1 -> Multiply/1, Subtract/2
  Subtract/1 -> Divide/1
  Add/1 -> Scope/1, Position (rad)/1
  Multiply/1 -> Subtract1/2
  Input(v)/1 -> Subtract/1
  Subtract1/1 -> Add/2
  Default Zero/1 -> Subtract1/1

== system PD_Diagonal/Control Allocation/M1/M1 Y Servo ==
  note: 0V Servo = 0 degree / +90 offset
      | 2.5v Servo = 90 degree/ 0 offset
      | 5v Servo = 180 degree / -90 offset
  note: Servo zero position = 2.5v = 90 degree vertical
  note: 2.5v = 90 degree
  note: 2.5v = 0 offset
  note: M1Y Servo Response v->rad
  Input(v) : Inport
  ->ms : Product  Inputs=*/
  ->rad : Constant  Value=pi/5
  Add : Sum  Inputs=+-
  Dead Time (ms) : Constant  Value=3
  Dead Time Block : VariableTransportDelay  MaximumDelay=10
  Default Zero : Constant  Value=pi/2
  Divide : Product  Inputs=*/
  Limits : Constant  OutDataTypeStr=boolean
  Miliseconds : Constant  Value=1000
  Multiply : Product  Inputs=**
  Saturation : Subsystem
  Scope : Scope
      settings: SaveName=ScopeData4
  Starting Position(v) : Constant  Value=2.5
  Subtract : Sum  Inputs=|-+
  Subtract1 : Sum  Inputs=+-|
  Supply (V) : Constant  Value=5
  Transfer Fcn : TransferFcn  Numerator=[pi]  Denominator=[0.11 1]
  Position (rad) : Outport
  wires:
  Miliseconds/1 -> ->ms/2
  Dead Time (ms)/1 -> ->ms/1
  Supply (V)/1 -> Divide/2
  Divide/1 -> Dead Time Block/1
  ->ms/1 -> Dead Time Block/2  "Deadtime 3ms (333hz digital)"
  Dead Time Block/1 -> Transfer Fcn/1
  ->rad/1 -> Multiply/2
  Transfer Fcn/1 -> Saturation/1(Rad)
  Saturation/1(Out1) -> Add/1
  Limits/1 -> Saturation/2(1/0)
  Starting Position(v)/1 -> Multiply/1, Subtract/2
  Subtract/1 -> Divide/1
  Add/1 -> Scope/1, Position (rad)/1
  Multiply/1 -> Subtract1/2
  Input(v)/1 -> Subtract/1
  Subtract1/1 -> Add/2
  Default Zero/1 -> Subtract1/1

== system PD_Diagonal/Control Allocation/M1/M1->B Transformation ==
  note: X->Y->Z Transformation Sequence M1->B
  X : Inport
  Y : Inport  Port=2
  "Z " : Inport  Port=3
  Quaternion Multiplication : aerolibutil/Quaternion Multiplication
  Quaternion Multiplication1 : aerolibutil/Quaternion Multiplication
  X Quaternion : Subsystem
  Y Quaternion : Subsystem
  Z Quaternion : Subsystem
  Q_m1 : Outport
  wires:
  X/1 -> X Quaternion/1(y(X Rad))
  "Z "/1 -> Z Quaternion/1(Z Rad)
  Y/1 -> Y Quaternion/1(h(Y Rad))
  Y Quaternion/1(Q_y) -> Quaternion Multiplication/2  "Qy"
  X Quaternion/1(Q_x) -> Quaternion Multiplication/1  "Qx"
  Quaternion Multiplication/1 -> Quaternion Multiplication1/1  "Qx*Qy"
  Z Quaternion/1(Q_z) -> Quaternion Multiplication1/2  "Qz"
  Quaternion Multiplication1/1 -> Q_m1/1  "Qx*Qy*Qz"

== system PD_Diagonal/Control Allocation/M1 Distibution/Degress to Volts ==
  X(rad) : Inport
  Y(rad) : Inport  Port=2
  *pi/5 : Constant  Value=pi/5
  0 Point : Constant  Value=2.5
  Sum1 : Sum  Inputs=|++
  Sum4 : Sum  Inputs=++|
  X/180*1 : Product  Inputs=*/
  Y/180*1 : Product  Inputs=*/
  X(V) : Outport
  Y(V) : Outport  Port=2
  wires:
  X(rad)/1 -> X/180*1/1  "X(rad)"
  Y(rad)/1 -> Y/180*1/1  "Y(rad)"
  Sum1/1 -> X(V)/1
  0 Point/1 -> Sum1/2, Sum4/1
  *pi/5/1 -> X/180*1/2, Y/180*1/2
  Sum4/1 -> Y(V)/1
  X/180*1/1 -> Sum1/1
  Y/180*1/1 -> Sum4/2

== system PD_Diagonal/Control Allocation/M1 Distibution/MotorSpeed ==
  F_in : Inport
  Divide : Product  Inputs=*/
  Force Coefficient CT : Constant  Value=0.000243
  Mins : Constant  Value=60
  Product : Product
  w^2 : Sqrt  SaturateOnIntegerOverflow=on
  |F| : Sqrt  SaturateOnIntegerOverflow=on
  |F|^2 : DotProduct  InputSameDT=on  OutDataTypeStr=Inherit: Inherit via internal rule
  RPM : Outport
  wires:
  w^2/1 -> Product/2
  Product/1 -> RPM/1  "RPM"
  Mins/1 -> Product/1
  Divide/1 -> w^2/1
  Force Coefficient CT/1 -> Divide/2
  F_in/1 -> |F|^2/2, |F|^2/1
  |F|^2/1 -> |F|/1
  |F|/1 -> Divide/1

== system PD_Diagonal/Control Allocation/M1 Distibution/Solve M1 XY ==
  Fx : Inport
  Fy : Inport  Port=2
  Fz : Inport  Port=3
  -Fx/Fz : Gain  Gain=-1
  Constant : Constant  Value=pi
  Dot Product : DotProduct  InputSameDT=on  OutDataTypeStr=Inherit: Inherit via internal rule
  F : Concatenate  NumInputs=3
  Fx/Fz : Product  Inputs=*/
  Fy/T : Product  Inputs=*/
  Sum : Sum  Inputs=|-+
  Switch : Switch  Criteria=u2 > Threshold
  T : Sqrt  Operator=signedSqrt  SaturateOnIntegerOverflow=on
  asin(Fy/T) : Trigonometry  Operator=asin
  atan(-Fx/Fz) : Trigonometry  Operator=atan
  X : Outport
  Y : Outport  Port=2
  wires:
  Fy/1 -> F/2, Fy/T/1
  Fx/1 -> Fx/Fz/1, F/1
  Fz/1 -> F/3, Switch/2, Fx/Fz/2  "Fz"
  F/1 -> Dot Product/2, Dot Product/1
  Dot Product/1 -> T/1
  T/1 -> Fy/T/2  "T"
  Fy/T/1 -> asin(Fy/T)/1
  Fx/Fz/1 -> -Fx/Fz/1
  -Fx/Fz/1 -> atan(-Fx/Fz)/1
  asin(Fy/T)/1 -> Switch/1, Sum/1  "X"
  Switch/1 -> X/1
  Sum/1 -> Switch/3
  Constant/1 -> Sum/2
  atan(-Fx/Fz)/1 -> Y/1

== system PD_Diagonal/Control Allocation/M2/M1 DC Motor ==
  note: M1 DC Motor response
  Set Speed(rpm) : Inport
  ->ms : Product  Inputs=*/
  10080 Max : Saturate  UpperLimit=10080  LowerLimit=-10080
  Add : Sum
  Dead Time (ms) : Constant
  Dead Time Block : VariableTransportDelay  MaximumDelay=10
  Miliseconds : Constant  Value=1000
  Starting Speed : Constant  Value=-10080
  Subtract : Sum  Inputs=+-
  Transfer Fcn : TransferFcn  Numerator=1  Denominator=[0.6 1]
  Speed (rpm) : Outport
  wires:
  Dead Time Block/1 -> Transfer Fcn/1
  Miliseconds/1 -> ->ms/2
  Dead Time (ms)/1 -> ->ms/1
  ->ms/1 -> Dead Time Block/2
  Transfer Fcn/1 -> 10080 Max/1
  Set Speed(rpm)/1 -> Subtract/1
  10080 Max/1 -> Add/1
  Add/1 -> Speed (rpm)/1
  Starting Speed/1 -> Subtract/2, Add/2
  Subtract/1 -> Dead Time Block/1

== system PD_Diagonal/Control Allocation/M2/M1 Speed to Thrust ==
  note: RPS to Thrust
  Speed(RPM) : Inport
  ->RPS : Product  Inputs=*/
  Force Coefficient CT : Constant  Value=0.000243
  M1 w^2 : Math  Operator=magnitude^2  SaturateOnIntegerOverflow=on
  Mins : Constant  Value=60
  Product : Product
  Thrust(N) : Outport
  wires:
  M1 w^2/1 -> Product/2
  ->RPS/1 -> M1 w^2/1
  Speed(RPM)/1 -> ->RPS/1
  Force Coefficient CT/1 -> Product/1
  Mins/1 -> ->RPS/2
  Product/1 -> Thrust(N)/1

== system PD_Diagonal/Control Allocation/M2/M1 X Servo  ==
  note: 0V Servo = 0 degree / +90 offset
      | 2.5v Servo = 90 degree/ 0 offset
      | 5v Servo = 180 degree / -90 offset
  note: Servo zero position = 2.5v = 90 degree vertical
  note: 2.5v = 90 degree
  note: 2.5v = 0 offset
  note: M1X Servo Response v->rad
  Input(v) : Inport
  ->ms : Product  Inputs=*/
  ->rad : Constant  Value=pi/5
  Add : Sum  Inputs=+-
  Dead Time (ms) : Constant  Value=3
  Dead Time Block : VariableTransportDelay  MaximumDelay=10
  Default Zero : Constant  Value=pi/2
  Divide : Product  Inputs=*/
  Limits : Constant  OutDataTypeStr=boolean
  Miliseconds : Constant  Value=1000
  Multiply : Product  Inputs=**
  Saturation : Subsystem
  Scope : Scope
      settings: SaveName=ScopeData3
  Starting Position(v) : Constant  Value=2.5
  Subtract : Sum  Inputs=|-+
  Subtract1 : Sum  Inputs=+-|
  Supply (V) : Constant  Value=5
  Transfer Fcn : TransferFcn  Numerator=[pi]  Denominator=[0.11 1]
  Position (rad) : Outport
  wires:
  Miliseconds/1 -> ->ms/2
  Dead Time (ms)/1 -> ->ms/1
  Supply (V)/1 -> Divide/2
  Divide/1 -> Dead Time Block/1
  ->ms/1 -> Dead Time Block/2  "Deadtime 3ms (333hz digital)"
  Dead Time Block/1 -> Transfer Fcn/1
  ->rad/1 -> Multiply/2
  Transfer Fcn/1 -> Saturation/1(Rad)
  Saturation/1(Out1) -> Add/1
  Limits/1 -> Saturation/2(1/0)
  Starting Position(v)/1 -> Multiply/1, Subtract/2
  Subtract/1 -> Divide/1
  Add/1 -> Scope/1, Position (rad)/1
  Multiply/1 -> Subtract1/2
  Input(v)/1 -> Subtract/1
  Subtract1/1 -> Add/2
  Default Zero/1 -> Subtract1/1

== system PD_Diagonal/Control Allocation/M2/M1 Y Servo ==
  note: 0V Servo = 0 degree / +90 offset
      | 2.5v Servo = 90 degree/ 0 offset
      | 5v Servo = 180 degree / -90 offset
  note: Servo zero position = 2.5v = 90 degree vertical
  note: 2.5v = 90 degree
  note: 2.5v = 0 offset
  note: M1Y Servo Response v->rad
  Input(v) : Inport
  ->ms : Product  Inputs=*/
  ->rad : Constant  Value=pi/5
  Add : Sum  Inputs=+-
  Dead Time (ms) : Constant  Value=3
  Dead Time Block : VariableTransportDelay  MaximumDelay=10
  Default Zero : Constant  Value=pi/2
  Divide : Product  Inputs=*/
  Limits : Constant  OutDataTypeStr=boolean
  Miliseconds : Constant  Value=1000
  Multiply : Product  Inputs=**
  Saturation : Subsystem
  Scope : Scope
      settings: SaveName=ScopeData4
  Starting Position(v) : Constant  Value=2.5
  Subtract : Sum  Inputs=|-+
  Subtract1 : Sum  Inputs=+-|
  Supply (V) : Constant  Value=5
  Transfer Fcn : TransferFcn  Numerator=[pi]  Denominator=[0.11 1]
  Position (rad) : Outport
  wires:
  Miliseconds/1 -> ->ms/2
  Dead Time (ms)/1 -> ->ms/1
  Supply (V)/1 -> Divide/2
  Divide/1 -> Dead Time Block/1
  ->ms/1 -> Dead Time Block/2  "Deadtime 3ms (333hz digital)"
  Dead Time Block/1 -> Transfer Fcn/1
  ->rad/1 -> Multiply/2
  Transfer Fcn/1 -> Saturation/1(Rad)
  Saturation/1(Out1) -> Add/1
  Limits/1 -> Saturation/2(1/0)
  Starting Position(v)/1 -> Multiply/1, Subtract/2
  Subtract/1 -> Divide/1
  Add/1 -> Scope/1, Position (rad)/1
  Multiply/1 -> Subtract1/2
  Input(v)/1 -> Subtract/1
  Subtract1/1 -> Add/2
  Default Zero/1 -> Subtract1/1

== system PD_Diagonal/Control Allocation/M2/M1->B Transformation ==
  note: X->Y->Z Transformation Sequence M1->B
  X : Inport
  Y : Inport  Port=2
  "Z " : Inport  Port=3
  Quaternion Multiplication : aerolibutil/Quaternion Multiplication
  Quaternion Multiplication1 : aerolibutil/Quaternion Multiplication
  X Quaternion : Subsystem
  Y Quaternion : Subsystem
  Z Quaternion : Subsystem
  Q_m1 : Outport
  wires:
  X/1 -> X Quaternion/1(y(X Rad))
  "Z "/1 -> Z Quaternion/1(Z Rad)
  Y/1 -> Y Quaternion/1(h(Y Rad))
  Y Quaternion/1(Q_y) -> Quaternion Multiplication/2  "Qy"
  X Quaternion/1(Q_x) -> Quaternion Multiplication/1  "Qx"
  Quaternion Multiplication/1 -> Quaternion Multiplication1/1  "Qx*Qy"
  Z Quaternion/1(Q_z) -> Quaternion Multiplication1/2  "Qz"
  Quaternion Multiplication1/1 -> Q_m1/1  "Qx*Qy*Qz"

== system PD_Diagonal/Control Allocation/M2 Distibution/Degress to Volts ==
  X(rad) : Inport
  Y(rad) : Inport  Port=2
  *pi/5 : Constant  Value=pi/5
  0 Point : Constant  Value=2.5
  Sum1 : Sum  Inputs=|++
  Sum4 : Sum  Inputs=++|
  X/180*1 : Product  Inputs=*/
  Y/180*1 : Product  Inputs=*/
  X(V) : Outport
  Y(V) : Outport  Port=2
  wires:
  X(rad)/1 -> X/180*1/1  "X(rad)"
  Y(rad)/1 -> Y/180*1/1  "Y(rad)"
  Sum1/1 -> X(V)/1
  0 Point/1 -> Sum1/2, Sum4/1
  *pi/5/1 -> X/180*1/2, Y/180*1/2
  Sum4/1 -> Y(V)/1
  X/180*1/1 -> Sum1/1
  Y/180*1/1 -> Sum4/2

== system PD_Diagonal/Control Allocation/M2 Distibution/MotorSpeed ==
  F_in : Inport
  Divide : Product  Inputs=*/
  Force Coefficient CT : Constant  Value=0.000243
  Mins : Constant  Value=60
  Product : Product
  w^2 : Sqrt  SaturateOnIntegerOverflow=on
  |F| : Sqrt  SaturateOnIntegerOverflow=on
  |F|^2 : DotProduct  InputSameDT=on  OutDataTypeStr=Inherit: Inherit via internal rule
  RPM : Outport
  wires:
  w^2/1 -> Product/2
  Product/1 -> RPM/1  "RPM"
  Mins/1 -> Product/1
  Divide/1 -> w^2/1
  Force Coefficient CT/1 -> Divide/2
  F_in/1 -> |F|^2/2, |F|^2/1
  |F|^2/1 -> |F|/1
  |F|/1 -> Divide/1

== system PD_Diagonal/Control Allocation/M2 Distibution/Solve M2 XY ==
  Fx : Inport
  Fy : Inport  Port=2
  Fz : Inport  Port=3
  Constant : Constant  Value=pi
  Dot Product : DotProduct  InputSameDT=on  OutDataTypeStr=Inherit: Inherit via internal rule
  F : Concatenate  NumInputs=3
  Fy/Fz : Product  Inputs=*/
  Fy/T : Product  Inputs=*/
  Gain : Gain  Gain=-1
  Gain1 : Gain  Gain=-1
  Sum : Sum  Inputs=|-+
  Switch : Switch  Criteria=u2 > Threshold
  T : Sqrt  Operator=signedSqrt  SaturateOnIntegerOverflow=on
  asin(Fy/T) : Trigonometry  Operator=asin
  atan(-Fx/Fz) : Trigonometry  Operator=atan
  X : Outport
  Y : Outport  Port=2
  wires:
  Fy/1 -> Fy/Fz/1, F/2
  Fx/1 -> F/1, Fy/T/1
  Fz/1 -> F/3, Switch/2, Fy/Fz/2  "Fz"
  F/1 -> Dot Product/2, Dot Product/1
  Dot Product/1 -> T/1
  T/1 -> Fy/T/2  "T"
  asin(Fy/T)/1 -> Switch/1, Sum/1  "X"
  Switch/1 -> X/1
  Sum/1 -> Switch/3
  Constant/1 -> Sum/2
  atan(-Fx/Fz)/1 -> Y/1
  Fy/T/1 -> Gain/1
  Gain/1 -> asin(Fy/T)/1
  Fy/Fz/1 -> Gain1/1
  Gain1/1 -> atan(-Fx/Fz)/1

== system PD_Diagonal/Control Allocation/M3/M1 DC Motor ==
  note: M1 DC Motor response
  Set Speed(rpm) : Inport
  ->ms : Product  Inputs=*/
  10080 Max : Saturate  UpperLimit=10080  LowerLimit=-10080
  Add : Sum
  Dead Time (ms) : Constant
  Dead Time Block : VariableTransportDelay  MaximumDelay=10
  Miliseconds : Constant  Value=1000
  Starting Speed : Constant  Value=10080
  Subtract : Sum  Inputs=+-
  Transfer Fcn : TransferFcn  Numerator=1  Denominator=[0.6 1]
  Speed (rpm) : Outport
  wires:
  Dead Time Block/1 -> Transfer Fcn/1
  Miliseconds/1 -> ->ms/2
  Dead Time (ms)/1 -> ->ms/1
  ->ms/1 -> Dead Time Block/2
  Transfer Fcn/1 -> 10080 Max/1
  Set Speed(rpm)/1 -> Subtract/1
  10080 Max/1 -> Add/1
  Add/1 -> Speed (rpm)/1
  Starting Speed/1 -> Subtract/2, Add/2
  Subtract/1 -> Dead Time Block/1

== system PD_Diagonal/Control Allocation/M3/M1 Speed to Thrust ==
  note: RPS to Thrust
  Speed(RPM) : Inport
  ->RPS : Product  Inputs=*/
  Force Coefficient CT : Constant  Value=0.000243
  M1 w^2 : Math  Operator=magnitude^2  SaturateOnIntegerOverflow=on
  Mins : Constant  Value=60
  Product : Product
  Thrust(N) : Outport
  wires:
  M1 w^2/1 -> Product/2
  ->RPS/1 -> M1 w^2/1
  Speed(RPM)/1 -> ->RPS/1
  Force Coefficient CT/1 -> Product/1
  Mins/1 -> ->RPS/2
  Product/1 -> Thrust(N)/1

== system PD_Diagonal/Control Allocation/M3/M1 X Servo  ==
  note: 0V Servo = 0 degree / +90 offset
      | 2.5v Servo = 90 degree/ 0 offset
      | 5v Servo = 180 degree / -90 offset
  note: Servo zero position = 2.5v = 90 degree vertical
  note: 2.5v = 90 degree
  note: 2.5v = 0 offset
  note: M1X Servo Response v->rad
  Input(v) : Inport
  ->ms : Product  Inputs=*/
  ->rad : Constant  Value=pi/5
  Add : Sum  Inputs=+-
  Dead Time (ms) : Constant  Value=3
  Dead Time Block : VariableTransportDelay  MaximumDelay=10
  Default Zero : Constant  Value=pi/2
  Divide : Product  Inputs=*/
  Limits : Constant  OutDataTypeStr=boolean
  Miliseconds : Constant  Value=1000
  Multiply : Product  Inputs=**
  Saturation : Subsystem
  Scope : Scope
      settings: SaveName=ScopeData3
  Starting Position(v) : Constant  Value=2.5
  Subtract : Sum  Inputs=|-+
  Subtract1 : Sum  Inputs=+-|
  Supply (V) : Constant  Value=5
  Transfer Fcn : TransferFcn  Numerator=[pi]  Denominator=[0.11 1]
  Position (rad) : Outport
  wires:
  Miliseconds/1 -> ->ms/2
  Dead Time (ms)/1 -> ->ms/1
  Supply (V)/1 -> Divide/2
  Divide/1 -> Dead Time Block/1
  ->ms/1 -> Dead Time Block/2  "Deadtime 3ms (333hz digital)"
  Dead Time Block/1 -> Transfer Fcn/1
  ->rad/1 -> Multiply/2
  Transfer Fcn/1 -> Saturation/1(Rad)
  Saturation/1(Out1) -> Add/1
  Limits/1 -> Saturation/2(1/0)
  Starting Position(v)/1 -> Multiply/1, Subtract/2
  Subtract/1 -> Divide/1
  Add/1 -> Scope/1, Position (rad)/1
  Multiply/1 -> Subtract1/2
  Input(v)/1 -> Subtract/1
  Subtract1/1 -> Add/2
  Default Zero/1 -> Subtract1/1

== system PD_Diagonal/Control Allocation/M3/M1 Y Servo ==
  note: 0V Servo = 0 degree / +90 offset
      | 2.5v Servo = 90 degree/ 0 offset
      | 5v Servo = 180 degree / -90 offset
  note: Servo zero position = 2.5v = 90 degree vertical
  note: 2.5v = 90 degree
  note: 2.5v = 0 offset
  note: M1Y Servo Response v->rad
  Input(v) : Inport
  ->ms : Product  Inputs=*/
  ->rad : Constant  Value=pi/5
  Add : Sum  Inputs=+-
  Dead Time (ms) : Constant  Value=3
  Dead Time Block : VariableTransportDelay  MaximumDelay=10
  Default Zero : Constant  Value=pi/2
  Divide : Product  Inputs=*/
  Limits : Constant  OutDataTypeStr=boolean
  Miliseconds : Constant  Value=1000
  Multiply : Product  Inputs=**
  Saturation : Subsystem
  Scope : Scope
      settings: SaveName=ScopeData4
  Starting Position(v) : Constant  Value=2.5
  Subtract : Sum  Inputs=|-+
  Subtract1 : Sum  Inputs=+-|
  Supply (V) : Constant  Value=5
  Transfer Fcn : TransferFcn  Numerator=[pi]  Denominator=[0.11 1]
  Position (rad) : Outport
  wires:
  Miliseconds/1 -> ->ms/2
  Dead Time (ms)/1 -> ->ms/1
  Supply (V)/1 -> Divide/2
  Divide/1 -> Dead Time Block/1
  ->ms/1 -> Dead Time Block/2  "Deadtime 3ms (333hz digital)"
  Dead Time Block/1 -> Transfer Fcn/1
  ->rad/1 -> Multiply/2
  Transfer Fcn/1 -> Saturation/1(Rad)
  Saturation/1(Out1) -> Add/1
  Limits/1 -> Saturation/2(1/0)
  Starting Position(v)/1 -> Multiply/1, Subtract/2
  Subtract/1 -> Divide/1
  Add/1 -> Scope/1, Position (rad)/1
  Multiply/1 -> Subtract1/2
  Input(v)/1 -> Subtract/1
  Subtract1/1 -> Add/2
  Default Zero/1 -> Subtract1/1

== system PD_Diagonal/Control Allocation/M3/M1->B Transformation ==
  note: X->Y->Z Transformation Sequence M1->B
  X : Inport
  Y : Inport  Port=2
  "Z " : Inport  Port=3
  Quaternion Multiplication : aerolibutil/Quaternion Multiplication
  Quaternion Multiplication1 : aerolibutil/Quaternion Multiplication
  X Quaternion : Subsystem
  Y Quaternion : Subsystem
  Z Quaternion : Subsystem
  Q_m1 : Outport
  wires:
  X/1 -> X Quaternion/1(y(X Rad))
  "Z "/1 -> Z Quaternion/1(Z Rad)
  Y/1 -> Y Quaternion/1(h(Y Rad))
  Y Quaternion/1(Q_y) -> Quaternion Multiplication/2  "Qy"
  X Quaternion/1(Q_x) -> Quaternion Multiplication/1  "Qx"
  Quaternion Multiplication/1 -> Quaternion Multiplication1/1  "Qx*Qy"
  Z Quaternion/1(Q_z) -> Quaternion Multiplication1/2  "Qz"
  Quaternion Multiplication1/1 -> Q_m1/1  "Qx*Qy*Qz"
